simulink model "Workshop_as_sim_part1"  (Simulink 9.3)
settings: Solver=ode1  StartTime=0.0  StopTime=inf  FixedStep=0.001  RelTol=1e-3  EnableMultiTasking=on
PostLoadFcn:
  | qc_set_target_type(getConfigSet(bdroot, 'QUARC Default Target Configuration'));
undefined symbols (not defined in the file or in its folder): HIL, qc_get_step_size
libraries: quarc_library x8, simulink x2
settings Model: Creator=DCrymble  LastModifiedBy=jxs210080  SimulationMode=external  ExtModeTrigDuration=50000
settings SolverCC: PositivePriorityOrder=on
settings DataIOCC: LimitDataPoints=on
settings OptimizationCC: ExpressionDepthLimit=2147483647  InitFltsAndDblsToZero=on  LifeSpan=auto
settings DebuggingCC: SaveWithParameterizedLinksMsg=none  SolverPrmCheckMsg=warning  MultiTaskDSMMsg=warning  MultiTaskCondExecSysMsg=none  StateNameClashWarn=warning
settings RTWCC: SystemTargetFile=quarc_win64.tlc  TemplateMakefile=quarc_default_tmf  Description=QUARC Win64 Target
settings STFCustomTargetCC: TargetPreCompLibLocation=C:\PROGRA~3\QUARC\lib\2019a\win64\release  ConcurrentExecutionCompliant=on  SystemTargetFile=quarc_win64.tlc
settings GRTTargetCC: TargetPreCompLibLocation=C:\PROGRA~3\QUARC\lib\2019a\win64\release  ParMdlRefBuildCompliant=off  CompOptLevelCompliant=off  MatFileLogging=off  CPPClassGenCompliant=off  UseToolchainInfoCompliant=off  ExtMode=on  ExtModeMexFile=quarc_comm

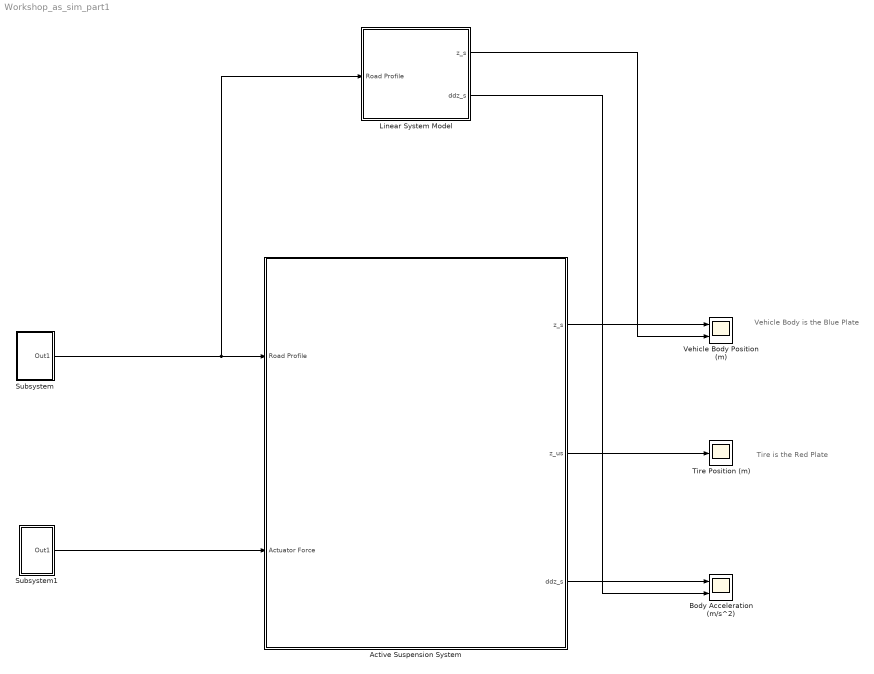
== system Workshop_as_sim_part1 ==
  note: Vehicle Body is the Blue Plate
  note: Tire is the Red Plate
  Active Suspension System : Subsystem
      mask Display: image('icon.png');
  Body Acceleration (m/s^2) : Scope  NumInputPorts=2
  Linear System Model : Subsystem
  Subsystem : Subsystem
  Subsystem1 : Subsystem
  Tire Position (m) : Scope
  Vehicle Body Position (m) : Scope  NumInputPorts=2
  wires:
  Active Suspension System/3(ddz_s) -> Body Acceleration (m/s^2)/1
  Active Suspension System/2(z_us) -> Tire Position (m)/1
  Active Suspension System/1(z_s) -> Vehicle Body Position (m)/1
  Subsystem1/1(Out1) -> Active Suspension System/2(Actuator Force)
  Subsystem/1(Out1) -> Linear System Model/1(Road Profile), Active Suspension System/1(Road Profile)
  Linear System Model/1(z_s) -> Vehicle Body Position (m)/2
  Linear System Model/2(ddz_s) -> Body Acceleration (m/s^2)/2

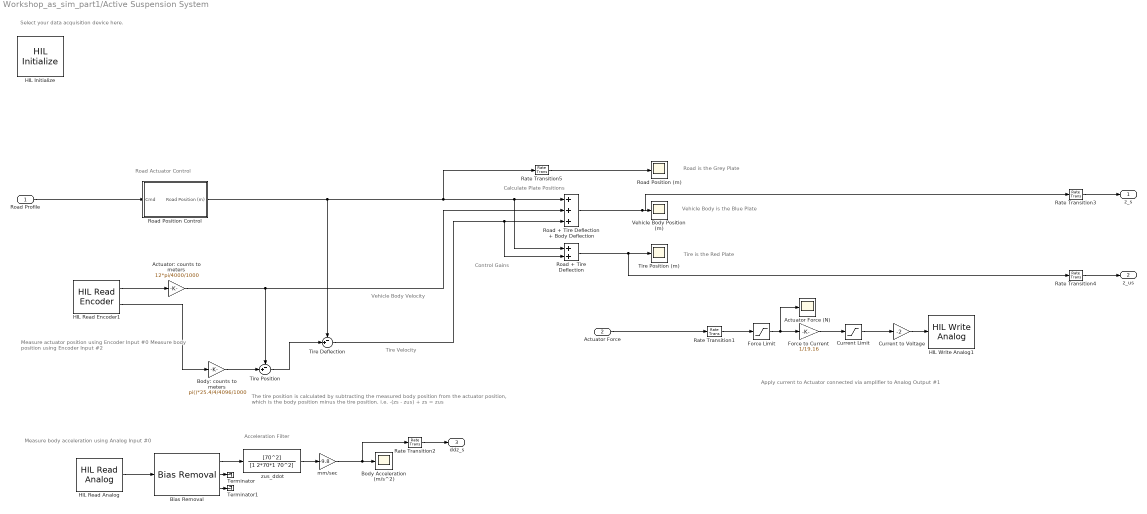
== system Workshop_as_sim_part1/Active Suspension System ==
  note: Measure actuator position using Encoder Input  #0
      | Measure body position using Encoder Input #2
  note: Select your data acquisition device here.
  note: Control Gains
  note: Vehicle Body Velocity
  note: Tire Velocity
  note: Road Actuator Control
  note: Calculate Plate Positions
  note: Measure body acceleration using Analog Input #0
  note: Acceleration Filter
  note: Apply current to Actuator connected via amplifier to Analog Output #1
  note: Road is the Grey Plate
  note: Vehicle Body is the Blue Plate
  note: Tire is the Red Plate
  note: The tire position is calculated by subtracting the measured body position from
      | the actuator position, which is the body position minus the tire position.
      | i.e. -(zs - zus) + zs = zus
  Road Profile : Inport
  Actuator Force : Inport  Port=2
  Actuator Force (N) : Scope
  Actuator: counts to meters : Gain  Gain=12*pi/4000/1000
  Bias Removal : quarc_library/Discrete/Bias Removal  start_time=0  end_time=.099  switch_id=0  sample_time=qc_get_step_size
      settings: SourceProductName=QUARC Targets
  Body Acceleration (m/s^2) : Scope
  Body: counts to meters : Gain  Gain=pi()*25.4/4/4096/1000
  Current Limit : Saturate  UpperLimit=5  LowerLimit=-5
  Current to Voltage : Gain  Gain=-2
  Force Limit : Saturate  UpperLimit=39.2  LowerLimit=-39.2
  Force to Current : Gain  Gain=1/19.16
  HIL Initialize : quarc_library/Data Acquisition/Generic/Configuration/HIL Initialize  Priority=-99  object_name=HIL-1  board_type=q8_usb  board_number=0  board_options=update_rate=normal;decimation=1  exclusive=off  active=off  hardware_clocks=[0:2]  clock_modes=[]  initial_clock_frequencies=[]  set_clock_params_at_start=off  set_clock_params_at_switch_in=off  set_clock_frequencies_at_start=off  set_clock_frequencies_at_switch_in=off  analog_input_channels=[0:7]  analog_input_configurations=[]  analog_input_maximums=10  analog_input_minimums=-10  set_analog_input_params_at_start=on  set_analog_input_params_at_switch_in=off  analog_output_channels=[0:7]  analog_output_maximums=10  analog_output_minimums=-10  initial_analog_outputs=[0]  final_analog_outputs=[0]  watchdog_analog_outputs=0  set_analog_output_params_at_start=on  set_analog_output_params_at_switch_in=off  set_analog_outputs_at_start=on  set_analog_outputs_at_switch_in=off  set_analog_outputs_at_terminate=on  set_analog_outputs_at_switch_out=off  set_analog_outputs_on_watchdog=off  digital_input_channels=[]  digital_output_channels=[0:4]  digital_output_configuration=[]  initial_digital_outputs=[0 0 0 0 1]  final_digital_outputs=[1 1 1 1 0]  watchdog_digital_outputs=[0]  set_digital_output_params_at_start=off  set_digital_output_params_at_switch_in=off  set_digital_outputs_at_start=on  set_digital_outputs_at_switch_in=on  set_digital_outputs_at_terminate=on  set_digital_outputs_at_switch_out=off  set_digital_outputs_on_watchdog=off  encoder_channels=[0:7]  quadrature=[4]  encoder_filter_frequency=[]  initial_encoder_counts=[0]  set_encoder_params_at_start=on  set_encoder_params_at_switch_in=off  set_encoder_counts_at_start=on  set_encoder_counts_at_switch_in=off  pwm_channels=[0:7]  pwm_modes=0  pwm_frequency=99.532799999999995e6/4095  pwm_configuration=[0]  pwm_alignment=[0]  pwm_polarity=[1]  pwm_leading_deadband=[0]  pwm_trailing_deadband=[0]  initial_pwm_outputs=[0]  final_pwm_outputs=[0]  watchdog_pwm_outputs=[0]  set_pwm_params_at_start=on  set_pwm_params_at_switch_in=off  set_pwm_outputs_at_start=on  set_pwm_outputs_at_switch_in=off  set_pwm_outputs_at_terminate=on  set_pwm_outputs_at_switch_out=off  set_pwm_outputs_on_watchdog=off  other_output_channels=[]  initial_other_outputs=[]  final_other_outputs=[]  watchdog_other_outputs=[]  set_other_outputs_at_start=off  set_other_outputs_at_switch_in=off  set_other_outputs_at_terminate=off  set_other_outputs_at_switch_out=off  set_other_outputs_on_watchdog=off
  HIL Read Analog : quarc_library/Data Acquisition/Generic/Immediate I//O/HIL Read Analog  object_name=HIL-1  channels=0  sample_time=qc_get_step_size  active=on  vector_output=off
  HIL Read Encoder1 : quarc_library/Data Acquisition/Generic/Immediate I//O/HIL Read Encoder  object_name=HIL-1  channels=[0, 2]  sample_time=qc_get_step_size  active=on  vector_output=off  data_type_mode=Inherit via back propagation  data_type=double
  HIL Write Analog1 : quarc_library/Data Acquisition/Generic/Immediate I//O/HIL Write Analog  object_name=HIL-1  channels=0  sample_time=-1  active=off  vector_input=on
  Rate Transition{1..5} (5 alike) : RateTransition  OutPortSampleTime=0.01
  Road + Tire Deflection : Sum  Inputs=2  SaturateOnIntegerOverflow=on  InputSameDT=on  OutDataTypeStr=Inherit: Same as first input
  Road + Tire Deflection + Body Deflection : Sum  Inputs=3  SaturateOnIntegerOverflow=on  InputSameDT=on  OutDataTypeStr=Inherit: Same as first input
  Road Position (m) : Scope
  Road Position Control : Subsystem
  Terminator : Terminator
  Terminator1 : Terminator
  Tire Deflection : Sum  Inputs=-+|
  Tire Position : Sum  Inputs=-+|
  Tire Position (m) : Scope
  Vehicle Body Position (m) : Scope
  mm/sec : Gain  Gain=-9.8
  zus_ddot : TransferFcn  Numerator=[70^2]  Denominator=[1 2*70*1 70^2]
  z_s : Outport
  z_us : Outport  Port=2
  ddz_s : Outport  Port=3
  wires:
  HIL Read Encoder1/1 -> Actuator: counts to meters/1
  Tire Deflection/1 -> Road + Tire Deflection + Body Deflection/3, Road + Tire Deflection/2
  HIL Read Encoder1/2 -> Body: counts to meters/1
  Body: counts to meters/1 -> Tire Position/2
  Road Position Control/1(Road Position (m)) -> Tire Deflection/1, Road + Tire Deflection + Body Deflection/1, Road + Tire Deflection/1, Rate Transition5/1
  Tire Position/1 -> Tire Deflection/2
  Bias Removal/2 -> Terminator/1
  Current to Voltage/1 -> HIL Write Analog1/1
  Force to Current/1 -> Current Limit/1
  Road Profile/1 -> Road Position Control/1(Cmd)
  Force Limit/1 -> Actuator Force (N)/1, Force to Current/1
  zus_ddot/1 -> mm/sec/1
  mm/sec/1 -> Rate Transition2/1, Body Acceleration (m/s^2)/1
  Bias Removal/1 -> zus_ddot/1
  Current Limit/1 -> Current to Voltage/1
  HIL Read Analog/1 -> Bias Removal/1
  Bias Removal/3 -> Terminator1/1
  Rate Transition2/1 -> ddz_s/1
  Rate Transition4/1 -> z_us/1
  Rate Transition3/1 -> z_s/1
  Rate Transition1/1 -> Force Limit/1
  Road + Tire Deflection + Body Deflection/1 -> Rate Transition3/1, Vehicle Body Position (m)/1
  Road + Tire Deflection/1 -> Rate Transition4/1, Tire Position (m)/1
  Actuator: counts to meters/1 -> Tire Position/1, Road + Tire Deflection + Body Deflection/2
  Rate Transition5/1 -> Road Position (m)/1
  Actuator Force/1 -> Rate Transition1/1

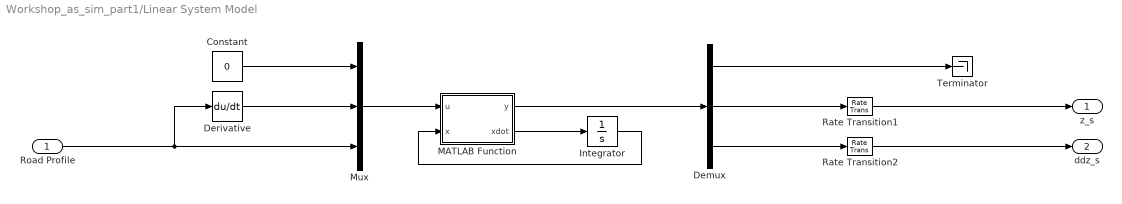
== system Workshop_as_sim_part1/Linear System Model ==
  Road Profile : Inport
  Constant : Constant  Value=0
  Demux : Demux  Outputs=3
  Derivative : Derivative
  Integrator : Integrator  InitialCondition=[-0.01;0;0.015;0]
  MATLAB Function : MATLAB Function  TreatAsAtomicUnit=on
  Mux : Mux  Inputs=3
  Rate Transition1 : RateTransition  OutPortSampleTime=0.01
  Rate Transition2 : RateTransition  OutPortSampleTime=0.01
  Terminator : Terminator
  z_s : Outport
  ddz_s : Outport  Port=2
  wires:
  Derivative/1 -> Mux/2
  Rate Transition2/1 -> ddz_s/1
  Constant/1 -> Mux/1
  Rate Transition1/1 -> z_s/1
  Demux/1 -> Terminator/1
  Demux/3 -> Rate Transition2/1
  Demux/2 -> Rate Transition1/1
  Integrator/1 -> MATLAB Function/2(x)
  MATLAB Function/2(xdot) -> Integrator/1
  Road Profile/1 -> Mux/3, Derivative/1
  Mux/1 -> MATLAB Function/1(u)
  MATLAB Function/1(y) -> Demux/1

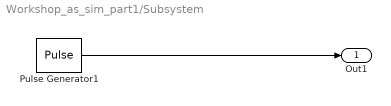
== system Workshop_as_sim_part1/Subsystem ==
  Pulse Generator1 : DiscretePulseGenerator  PulseType=Time based  Amplitude=0.02  Period=3  PulseWidth=50  PhaseDelay=.1
  Out1 : Outport
  wires:
  Pulse Generator1/1 -> Out1/1

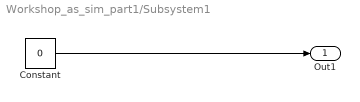
== system Workshop_as_sim_part1/Subsystem1 ==
  Constant : Constant  Value=0
  Out1 : Outport
  wires:
  Constant/1 -> Out1/1

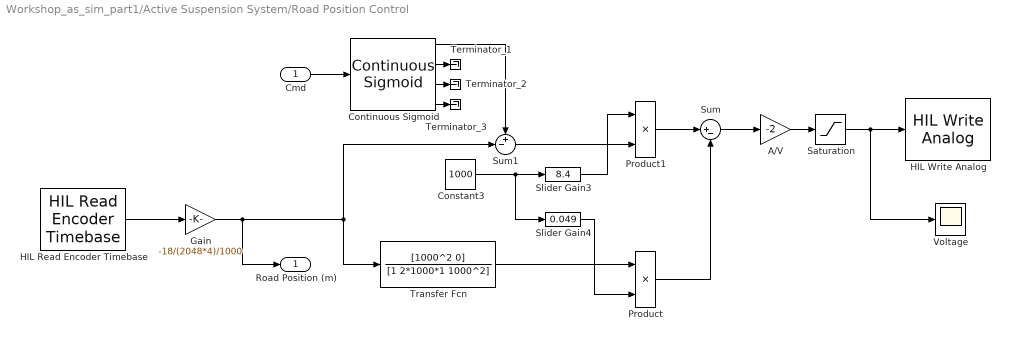
== system Workshop_as_sim_part1/Active Suspension System/Road Position Control ==
  Cmd : Inport
  A/V : Gain  Gain=-2
  Constant3 : Constant  Value=1000
  Continuous Sigmoid : quarc_library/Sources/Sigmoids/Continuous Sigmoid  params_source=Internal (dialog parameters)  max_velocity=.6/3  max_acceleration=20  initial_position=0  initial_velocity=0  hold_off=0.5  input_sample_time=-1  output_sample_time=qc_get_step_size
      settings: SourceProductName=QUARC Targets
  Gain : Gain  Gain=-18/(2048*4)/1000
  HIL Read Encoder Timebase : quarc_library/Data Acquisition/Generic/Timebases/HIL Read Encoder Timebase  object_name=HIL-1  clock=[0]  channels=1  samples_in_buffer=max(ceil(1/qc_get_step_size), 1)  active=on  vector_output=on  data_type_mode=Inherit via back propagation  data_type=double
  HIL Write Analog : quarc_library/Data Acquisition/Generic/Immediate I//O/HIL Write Analog  object_name=HIL-1  channels=1  sample_time=-1  active=off  vector_input=on
  Product : Product  RndMeth=Zero
  Product1 : Product  RndMeth=Zero
  Saturation : Saturate  UpperLimit=10  LowerLimit=-10
  Slider Gain3 : simulink/Math Operations/Slider Gain  gain=8.4  low=0  high=70
  Slider Gain4 : simulink/Math Operations/Slider Gain  gain=0.049  low=0  high=0.1
  Sum : Sum  Inputs=|+-
  Sum1 : Sum  Inputs=+-|
  Terminator_1 : Terminator
  Terminator_2 : Terminator
  Terminator_3 : Terminator
  Transfer Fcn : TransferFcn  Numerator=[1000^2 0]  Denominator=[1 2*1000*1 1000^2]
  Voltage : Scope
  Road Position (m) : Outport
  wires:
  A/V/1 -> Saturation/1
  Constant3/1 -> Slider Gain4/1, Slider Gain3/1
  HIL Read Encoder Timebase/1 -> Gain/1
  Saturation/1 -> HIL Write Analog/1, Voltage/1
  Sum/1 -> A/V/1
  Gain/1 -> Road Position (m)/1, Transfer Fcn/1, Sum1/2
  Transfer Fcn/1 -> Product/1
  Slider Gain3/1 -> Product1/1
  Sum1/1 -> Product1/2
  Product1/1 -> Sum/1
  Slider Gain4/1 -> Product/2
  Product/1 -> Sum/2
  Continuous Sigmoid/2 -> Terminator_1/1
  Continuous Sigmoid/3 -> Terminator_2/1
  Continuous Sigmoid/4 -> Terminator_3/1
  Continuous Sigmoid/1 -> Sum1/1
  Cmd/1 -> Continuous Sigmoid/1

== matlab function Linear System Model/MATLAB Function ==
  data: u input double; x input double; y output double; xdot output double
function [y,xdot] = fcn(u,x)

% System dimensions
nx = 4; % Number of states
nu = 1; % Number of inputs (controllable)
nd = 2; % Number of disturbances
ny = 3; % Number of outputs

% Model parameters
Ks = 900;    % Suspension Stiffness (N/m) 
Kus = 1250;  % Tire stiffness (N/m)
Ms = 2.45;   % Sprung Mass (kg) 
Mus = 1;     % Unsprung Mass (kg)
Bs = 7.5;    % Suspension Inherent Damping coefficient (sec/m)
Bus = 5;     % Tire Inherent Damping coefficient (sec/m)

% Model Definition
Ac = [0 1 0 0
      -(Kus/Mus) -(Bs +Bus)/Mus (Ks/Mus) (Bs/Mus)
      0 -1 0 1
      0 (Bs/Ms) -(Ks/Ms) -(Bs/Ms)];   % State Matrix
Bc = [0; -(1/Mus); 0; (1/Ms)];        % Input Matrix
Vc = [-1 0
      (Bus/Mus) 0
      0 0
      0 0];                           % Disturbance
C = [1 0 0 0
     1 0 1 0
     0 (Bs/Ms) -(Ks/Ms) -(Bs/Ms)];    % Output
D = [0;0;(1/Ms)];                     % Feed-through
W = [0 1
     0 1
     0 0];                            % Output Disturbance


A = Ac;
B = [Bc Vc];
C = C;
D = [D W];



xdot = A*x + B*u;
y = C*x+D*u;
